simulink model "gocq0"  (R2019a)
settings: Solver=VariableStepAuto  StartTime=0.0  StopTime=10.0  RelTol=1e-3
settings Model: Creator=dell  LastModifiedBy=dell

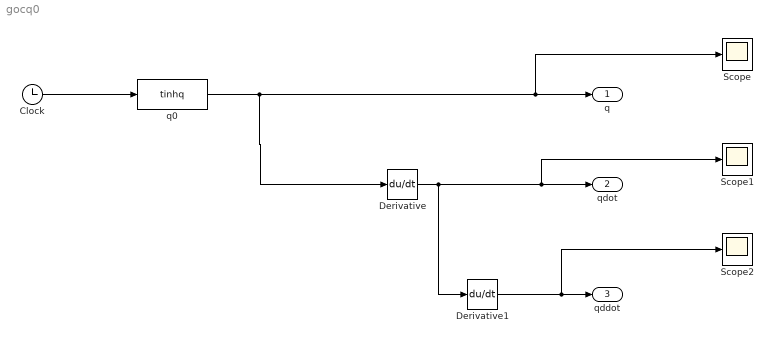
== system gocq0 ==
  Clock : Clock
      settings: Decimation=3
  Derivative : Derivative
  Derivative1 : Derivative
  Scope : Scope
  Scope1 : Scope
  Scope2 : Scope
  q0 : MATLABFcn  MATLABFcn=tinhq
  q : Outport
  qdot : Outport  Port=2
  qddot : Outport  Port=3
  wires:
  q0/1 -> q/1, Scope/1, Derivative/1
  Derivative1/1 -> Scope2/1, qddot/1
  Clock/1 -> q0/1
  Derivative/1 -> Derivative1/1, Scope1/1, qdot/1
